simulink model "bao2"  (R2018b)
settings: Solver=FixedStepAuto  StartTime=0.0  StopTime=50  FixedStep=0.005  RelTol=1e-3
settings Model: Creator=User  LastModifiedBy=User
settings SolverCC: AlgebraicLoopSolver=LineSearch

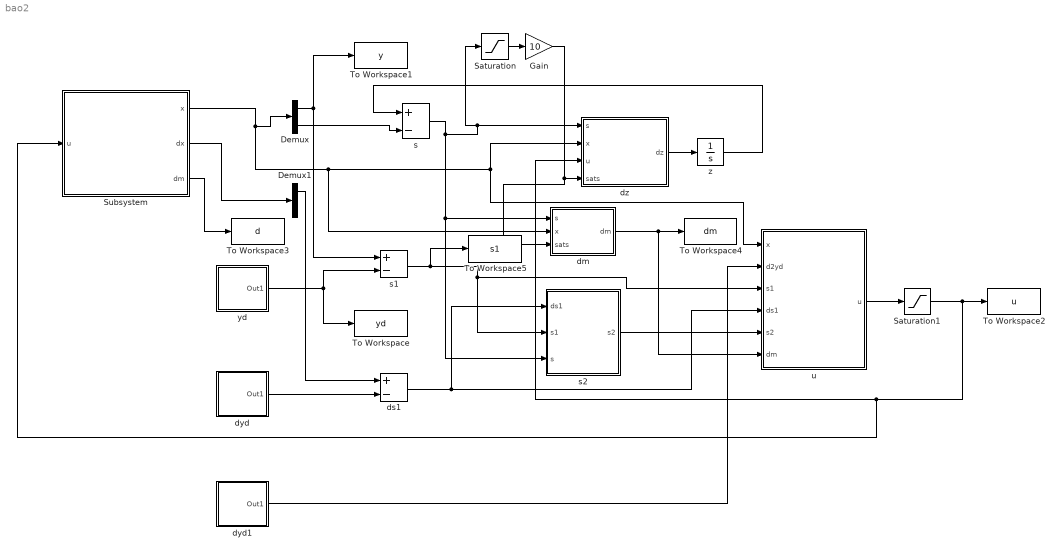
== system bao2 ==
  Demux : Demux  Outputs=2
  Demux1 : Demux  Outputs=2
  Gain : Gain  Gain=10
  Saturation : Saturate  UpperLimit=0.1  LowerLimit=-0.1
  Saturation1 : Saturate  UpperLimit=6  LowerLimit=-8
  Subsystem : Subsystem
  To Workspace : ToWorkspace  VariableName=yd  SampleTime=-1
  To Workspace1 : ToWorkspace  VariableName=y  SampleTime=-1
  To Workspace2 : ToWorkspace  VariableName=u  SampleTime=-1
  To Workspace3 : ToWorkspace  VariableName=d  SampleTime=-1
  To Workspace4 : ToWorkspace  VariableName=dm  SampleTime=-1
  To Workspace5 : ToWorkspace  VariableName=s1  SampleTime=-1
  dm : MATLAB Function  TreatAsAtomicUnit=on
  ds1 : Sum  Inputs=+-
  dyd : Subsystem
  dyd1 : Subsystem
  dz : MATLAB Function  TreatAsAtomicUnit=on
  s : Sum  Inputs=+-
  s1 : Sum  Inputs=+-
  s2 : MATLAB Function  TreatAsAtomicUnit=on
  u : MATLAB Function  TreatAsAtomicUnit=on
  yd : Subsystem
  z : Integrator  InitialCondition=0.2
  wires:
  Subsystem/1(x) -> dm/2(x), u/1(x), dz/2(x), Demux/1
  Demux/2 -> s/2
  dz/1(dz) -> z/1
  z/1 -> s/1
  dm/1(dm) -> To Workspace4/1, u/6(dm)
  s/1 -> Saturation/1, dz/1(s), s2/3(s), dm/1(s)
  Saturation/1 -> Gain/1
  Gain/1 -> dm/3(sats), dz/4(sats)
  Subsystem/3(dm) -> To Workspace3/1
  yd/1(Out1) -> To Workspace/1, s1/2
  Demux/1 -> s1/1, To Workspace1/1
  s1/1 -> To Workspace5/1, u/3(s1), s2/2(s1)
  dyd/1(Out1) -> ds1/2
  Subsystem/2(dx) -> Demux1/1
  Demux1/1 -> ds1/1
  ds1/1 -> u/4(ds1), s2/1(ds1)
  s2/1(s2) -> u/5(s2)
  dyd1/1(Out1) -> u/2(d2yd)
  u/1(u) -> Saturation1/1
  Saturation1/1 -> To Workspace2/1, Subsystem/1(u), dz/3(u)

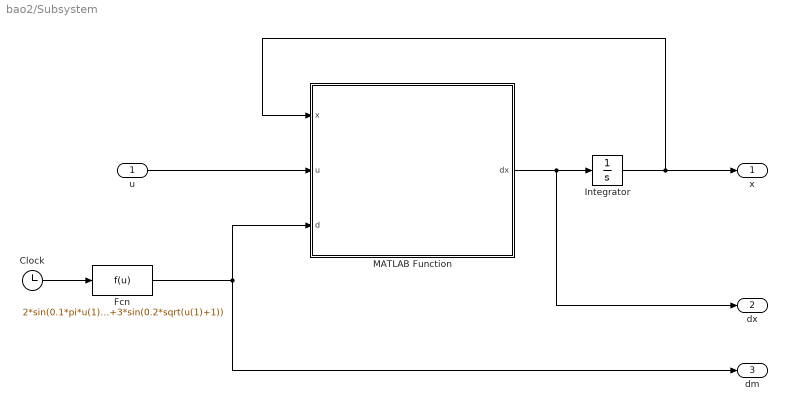
== system bao2/Subsystem ==
  u : Inport
  Clock : Clock
  Fcn : Fcn  Expr=2*sin(0.1*pi*u(1))+3*sin(0.2*sqrt(u(1)+1))
  Integrator : Integrator  InitialCondition=[0.1;0.2]
  MATLAB Function : MATLAB Function  TreatAsAtomicUnit=on
  x : Outport
  dx : Outport  Port=2
  dm : Outport  Port=3
  wires:
  Fcn/1 -> MATLAB Function/3(d), dm/1
  Clock/1 -> Fcn/1
  Integrator/1 -> x/1, MATLAB Function/1(x)
  MATLAB Function/1(dx) -> dx/1, Integrator/1
  u/1 -> MATLAB Function/2(u)

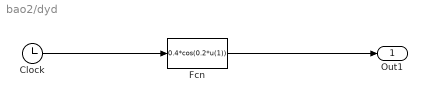
== system bao2/dyd ==
  Clock : Clock
  Fcn : Fcn  Expr=0.4*cos(0.2*u(1))
  Out1 : Outport
  wires:
  Clock/1 -> Fcn/1
  Fcn/1 -> Out1/1

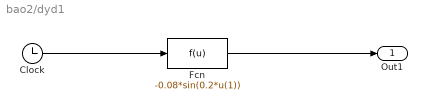
== system bao2/dyd1 ==
  Clock : Clock
  Fcn : Fcn  Expr=-0.08*sin(0.2*u(1))
  Out1 : Outport
  wires:
  Fcn/1 -> Out1/1
  Clock/1 -> Fcn/1

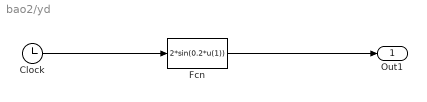
== system bao2/yd ==
  Clock : Clock
  Fcn : Fcn  Expr=2*sin(0.2*u(1))
  Out1 : Outport
  wires:
  Fcn/1 -> Out1/1
  Clock/1 -> Fcn/1

== matlab function bao2/dz ==
  data: s input; x input; u input; dz output; sats input
function dz = fcn(s,x,u,sats)
k=25;
beta=5;
eps=0.5;
p0=5;
q0=9;
dz=-k*s-beta*sats-eps*nthroot(s^p0,q0)-abs(-2*x(1)+3*(1-x(1)^2)*x(2))*sats+u;
end

== matlab function bao2/Subsystem/MATLAB Function ==
  data: x input; u input; dx output; d input
function dx = fcn(x,u,d)
dx=[x(2);
    -2*x(1)+3*(1-x(1)^2)*x(2)+u+d];
end

== matlab function bao2/s2 ==
  data: ds1 input; s2 output; s1 input; s input
function s2 = fcn(ds1,s1,s)
alp1=50;
bet1=0.5;
p1=5;
q1=7;
s2=ds1+alp1*s1+bet1*abs(s1)^(p1/q1)*sign(s1)+s;
end

== matlab function bao2/dm ==
  data: s input; x input; dm output; sats input
function dm = fcn(s,x,sats)
k=25;
beta=5;
eps=0.5;
p0=5;
q0=9;
dm=-k*s-beta*sats-eps*abs(s)^(p0/q0)*sign(s)-abs(-2*x(1)+3*(1-x(1)^2)*x(2))*sats+2*x(1)-3*(1-x(1)^2)*x(2);
end

== matlab function bao2/u ==
  data: x input; u output; d2yd input; s1 input; ds1 input; s2 input; dm input
function u = fcn(x,d2yd,s1,ds1,s2,dm)                           
alp1=50;
bet1=0.5;
p1=5;
q1=7;
p2=5;
q2=7;
del=60;
muy=0.8;
u=2*x(1)-3*(1-x(1)^2)*x(2)+d2yd-alp1*ds1-bet1*p1/q1*abs(s1)^(p1/q1-1)*ds1-dm-del*s2-muy*abs(s2)^(p2/q2)*sign(s2);
end
